simulink library "ovr"  (Simulink 8.2)
settings: Solver=ode45  StartTime=0.0  StopTime=10.0  RelTol=1e-3
undefined symbols (not defined in the file or in its folder): AIFO_HMIVehSpd_mps, C_TICK_TIME_S, ENUM_HMISTATE_ACTIVE, FALSE, KIFO_DriverOverrideTimer_ms, KIFO_ThrottleOverrideLimit_pct, KIFO_ThrottlePosTimeDelay_ms, KIFO_ThrottleVariationOvr_pctps, MIFO_HMISteerAngleLimit_deg, MIFO_HMISteerSpeedLimit_degps, TRUE
libraries: hcu_lib x2, simulink x1, idiada_lib x1
settings Model: Creator=xsellart  LastModifiedBy=14069

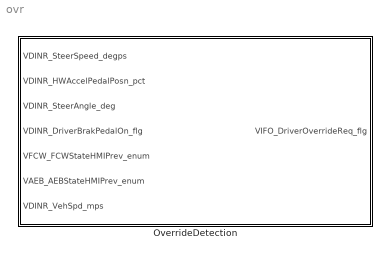
== system ovr ==
  OverrideDetection : Subsystem

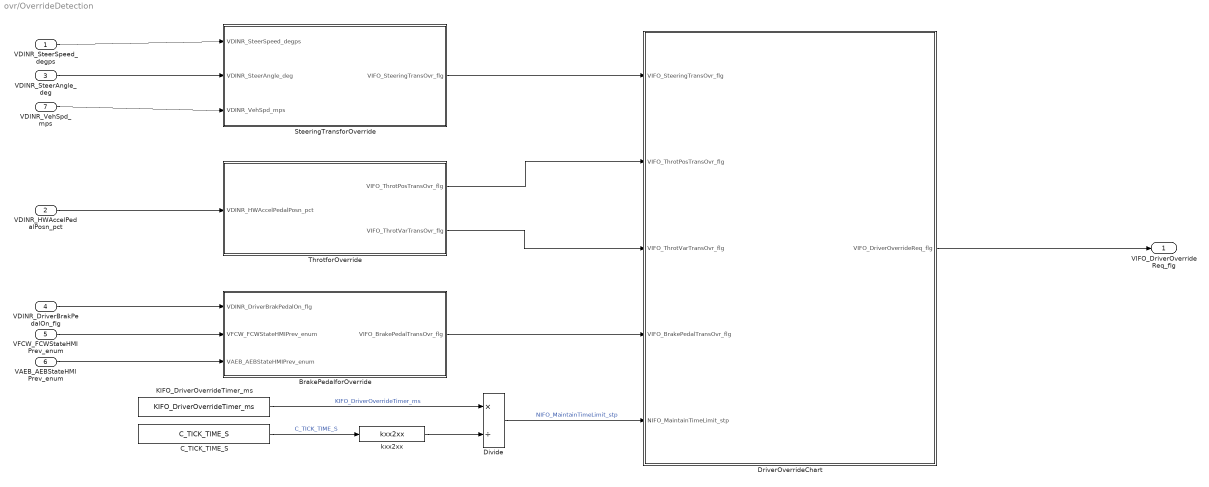
== system ovr/OverrideDetection ==
  VDINR_SteerSpeed_degps : Inport
  VDINR_HWAccelPedalPosn_pct : Inport  Port=2
  VDINR_SteerAngle_deg : Inport  Port=3
  VDINR_DriverBrakPedalOn_flg : Inport  Port=4
  VFCW_FCWStateHMIPrev_enum : Inport  Port=5
  VAEB_AEBStateHMIPrev_enum : Inport  Port=6
  VDINR_VehSpd_mps : Inport  Port=7
  BrakePedalforOverride : Subsystem
  C_TICK_TIME_S : Constant  Value=C_TICK_TIME_S  OutDataTypeStr=single
  Divide : Product  Inputs=*/
  DriverOverrideChart : Stateflow chart  TreatAsAtomicUnit=on
  KIFO_DriverOverrideTimer_ms : Constant  Value=KIFO_DriverOverrideTimer_ms  OutDataTypeStr=single
  SteeringTransforOverride : Subsystem
  ThrotforOverride : Subsystem
  kxx2xx : hcu_lib/kxx2xx
  VIFO_DriverOverrideReq_flg : Outport
  wires:
  kxx2xx/1 -> Divide/2
  Divide/1 -> DriverOverrideChart/5(NIFO_MaintainTimeLimit_stp)  "NIFO_MaintainTimeLimit_stp"
  C_TICK_TIME_S/1 -> kxx2xx/1  "C_TICK_TIME_S"
  KIFO_DriverOverrideTimer_ms/1 -> Divide/1  "KIFO_DriverOverrideTimer_ms"
  VDINR_DriverBrakPedalOn_flg/1 -> BrakePedalforOverride/1(VDINR_DriverBrakPedalOn_flg)
  VFCW_FCWStateHMIPrev_enum/1 -> BrakePedalforOverride/2(VFCW_FCWStateHMIPrev_enum)
  BrakePedalforOverride/1(VIFO_BrakePedalTransOvr_flg) -> DriverOverrideChart/4(VIFO_BrakePedalTransOvr_flg)
  VAEB_AEBStateHMIPrev_enum/1 -> BrakePedalforOverride/3(VAEB_AEBStateHMIPrev_enum)
  ThrotforOverride/2(VIFO_ThrotVarTransOvr_flg) -> DriverOverrideChart/3(VIFO_ThrotVarTransOvr_flg)
  ThrotforOverride/1(VIFO_ThrotPosTransOvr_flg) -> DriverOverrideChart/2(VIFO_ThrotPosTransOvr_flg)
  VDINR_HWAccelPedalPosn_pct/1 -> ThrotforOverride/1(VDINR_HWAccelPedalPosn_pct)
  SteeringTransforOverride/1(VIFO_SteeringTransOvr_flg) -> DriverOverrideChart/1(VIFO_SteeringTransOvr_flg)
  VDINR_SteerAngle_deg/1 -> SteeringTransforOverride/2("VDINR_SteerAngle_deg ")
  VDINR_SteerSpeed_degps/1 -> SteeringTransforOverride/1(VDINR_SteerSpeed_degps)
  DriverOverrideChart/1(VIFO_DriverOverrideReq_flg) -> VIFO_DriverOverrideReq_flg/1
  VDINR_VehSpd_mps/1 -> SteeringTransforOverride/3(VDINR_VehSpd_mps)

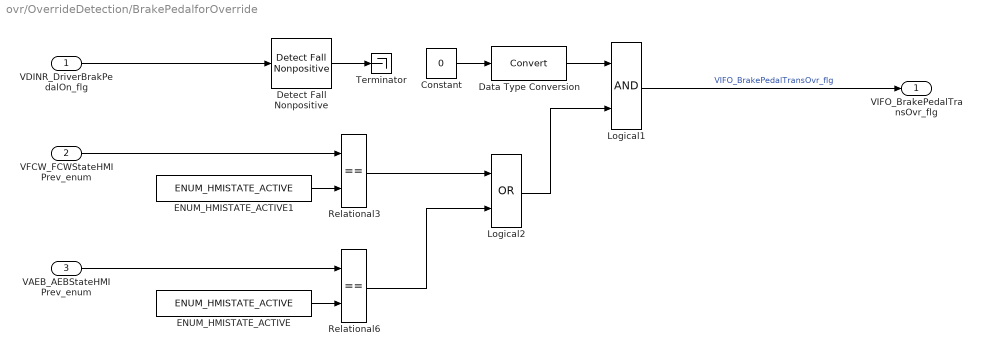
== system ovr/OverrideDetection/BrakePedalforOverride ==
  VDINR_DriverBrakPedalOn_flg : Inport
  VFCW_FCWStateHMIPrev_enum : Inport  Port=2
  VAEB_AEBStateHMIPrev_enum : Inport  Port=3
  Constant : Constant  Value=0
  Data Type Conversion : DataTypeConversion
  Detect Fall Nonpositive : simulink/Logic and Bit Operations/Detect Fall Nonpositive  vinit=0  InputProcessing=Inherited  OutDataTypeStr=boolean
  ENUM_HMISTATE_ACTIVE : Constant  Value=ENUM_HMISTATE_ACTIVE
  ENUM_HMISTATE_ACTIVE1 : Constant  Value=ENUM_HMISTATE_ACTIVE  OutDataTypeStr=uint8
  Logical1 : Logic  AllPortsSameDT=off  OutDataTypeStr=boolean
  Logical2 : Logic  Operator=OR  AllPortsSameDT=off  OutDataTypeStr=boolean
  Relational3 : RelationalOperator  Operator===  OutDataTypeStr=boolean
  Relational6 : RelationalOperator  Operator===  OutDataTypeStr=boolean
  Terminator : Terminator
  VIFO_BrakePedalTransOvr_flg : Outport
  wires:
  Logical2/1 -> Logical1/2
  Logical1/1 -> VIFO_BrakePedalTransOvr_flg/1  "VIFO_BrakePedalTransOvr_flg"
  Relational6/1 -> Logical2/2
  Relational3/1 -> Logical2/1
  ENUM_HMISTATE_ACTIVE/1 -> Relational6/2
  VAEB_AEBStateHMIPrev_enum/1 -> Relational6/1
  ENUM_HMISTATE_ACTIVE1/1 -> Relational3/2
  VFCW_FCWStateHMIPrev_enum/1 -> Relational3/1
  Detect Fall Nonpositive/1 -> Terminator/1
  VDINR_DriverBrakPedalOn_flg/1 -> Detect Fall Nonpositive/1
  Constant/1 -> Data Type Conversion/1
  Data Type Conversion/1 -> Logical1/1

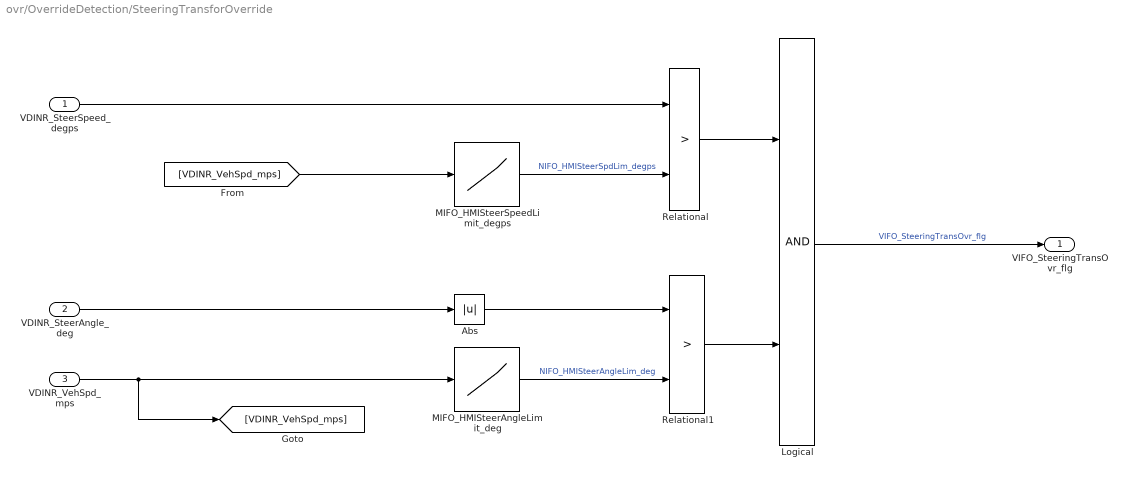
== system ovr/OverrideDetection/SteeringTransforOverride ==
  VDINR_SteerSpeed_degps : Inport
  "VDINR_SteerAngle_deg " : Inport  Port=2
  VDINR_VehSpd_mps : Inport  Port=3
  Abs : Abs
  Logical : Logic  AllPortsSameDT=off  OutDataTypeStr=boolean
  MIFO_HMISteerAngleLimit_deg : Lookup_n-D  NumberOfTableDimensions=1  BreakpointsForDimension1=AIFO_HMIVehSpd_mps  Table=MIFO_HMISteerAngleLimit_deg  RndMeth=Simplest  InputSameDT=on
  MIFO_HMISteerSpeedLimit_degps : Lookup_n-D  NumberOfTableDimensions=1  BreakpointsForDimension1=AIFO_HMIVehSpd_mps  Table=MIFO_HMISteerSpeedLimit_degps  RndMeth=Simplest  InputSameDT=on
  Relational : RelationalOperator  Operator=>  OutDataTypeStr=boolean
  Relational1 : RelationalOperator  Operator=>  OutDataTypeStr=boolean
  VIFO_SteeringTransOvr_flg : Outport
  wires:
  Abs/1 -> Relational1/1
  VDINR_SteerSpeed_degps/1 -> Relational/1
  "VDINR_SteerAngle_deg "/1 -> Abs/1
  Relational1/1 -> Logical/2
  Relational/1 -> Logical/1
  Logical/1 -> VIFO_SteeringTransOvr_flg/1  "VIFO_SteeringTransOvr_flg"
  MIFO_HMISteerAngleLimit_deg/1 -> Relational1/2  "NIFO_HMISteerAngleLim_deg"
  MIFO_HMISteerSpeedLimit_degps/1 -> Relational/2  "NIFO_HMISteerSpdLim_degps"
  [VDINR_VehSpd_mps] -> MIFO_HMISteerSpeedLimit_degps/1
  VDINR_VehSpd_mps/1 -> [VDINR_VehSpd_mps], MIFO_HMISteerAngleLimit_deg/1

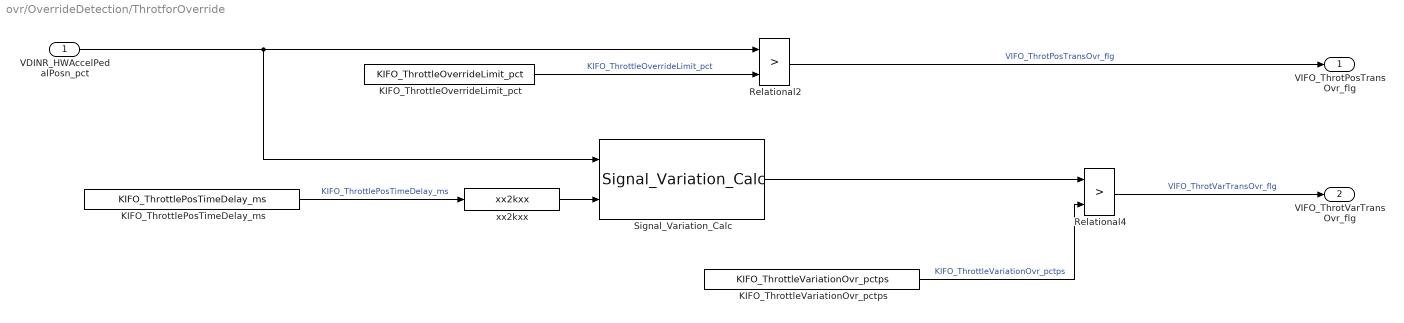
== system ovr/OverrideDetection/ThrotforOverride ==
  VDINR_HWAccelPedalPosn_pct : Inport
  KIFO_ThrottleOverrideLimit_pct : Constant  Value=KIFO_ThrottleOverrideLimit_pct  OutDataTypeStr=single
  KIFO_ThrottlePosTimeDelay_ms : Constant  Value=KIFO_ThrottlePosTimeDelay_ms
  KIFO_ThrottleVariationOvr_pctps : Constant  Value=KIFO_ThrottleVariationOvr_pctps  OutDataTypeStr=single
  Relational2 : RelationalOperator  Operator=>  OutDataTypeStr=boolean
  Relational4 : RelationalOperator  Operator=>  OutDataTypeStr=boolean
  Signal_Variation_Calc : idiada_lib/Signal_Variation_Calc
  xx2kxx : hcu_lib/xx2kxx
  VIFO_ThrotPosTransOvr_flg : Outport
  VIFO_ThrotVarTransOvr_flg : Outport  Port=2
  wires:
  xx2kxx/1 -> Signal_Variation_Calc/2
  Signal_Variation_Calc/1 -> Relational4/1
  KIFO_ThrottlePosTimeDelay_ms/1 -> xx2kxx/1  "KIFO_ThrottlePosTimeDelay_ms"
  Relational4/1 -> VIFO_ThrotVarTransOvr_flg/1  "VIFO_ThrotVarTransOvr_flg"
  KIFO_ThrottleVariationOvr_pctps/1 -> Relational4/2  "KIFO_ThrottleVariationOvr_pctps"
  KIFO_ThrottleOverrideLimit_pct/1 -> Relational2/2  "KIFO_ThrottleOverrideLimit_pct"
  VDINR_HWAccelPedalPosn_pct/1 -> Relational2/1, Signal_Variation_Calc/1
  Relational2/1 -> VIFO_ThrotPosTransOvr_flg/1  "VIFO_ThrotPosTransOvr_flg"

== stateflow chart OverrideDetection/DriverOverrideChart ==
  state OFF
    en:
    VIFO_DriverOverrideReq_flg = FALSE;
  state ON
    en:
    VIFO_DriverOverrideReq_flg = TRUE;
  state MAINTAIN
    en:
    NIFO_MaintainTimeLocal_stp = 0;
    du:
    NIFO_MaintainTimeLocal_stp=NIFO_MaintainTimeLocal_stp+1;
  (default) -> OFF
  ON -> MAINTAIN : [VIFO_SteeringTransOvr_flg==FALSE...
      | && VIFO_ThrotPosTransOvr_flg==FALSE]
  OFF -> ON : [VIFO_SteeringTransOvr_flg==TRUE...
      | || VIFO_ThrotPosTransOvr_flg==TRUE...
      | || VIFO_ThrotVarTransOvr_flg==TRUE...
      | || VIFO_BrakePedalTransOvr_flg == TRUE]
  MAINTAIN -> ON [order 1] : [VIFO_SteeringTransOvr_flg==TRUE...
      | || VIFO_ThrotPosTransOvr_flg==TRUE...
      | || VIFO_ThrotVarTransOvr_flg==TRUE]
  MAINTAIN -> (junction 16) [order 2]
  (junction 15) -> OFF
  (junction 16) -> (junction 15) : [NIFO_MaintainTimeLocal_stp>NIFO_MaintainTimeLimit_stp]
  data: VIFO_DriverOverrideReq_flg output boolean; VIFO_SteeringTransOvr_flg input boolean; VIFO_ThrotPosTransOvr_flg input boolean; VIFO_ThrotVarTransOvr_flg input boolean; FALSE parameter double; TRUE parameter double; VIFO_BrakePedalTransOvr_flg input boolean; NIFO_MaintainTimeLocal_stp local single; NIFO_MaintainTimeLimit_stp input single
